simulink model "weight_update"  (R2020a)
settings: Solver=VariableStepAuto  StartTime=0.0  StopTime=6  RelTol=1e-3
libraries: fl_lib x23, ee_lib x10, nesl_utility x7
settings Model: Creator=nick  LastModifiedBy=nick

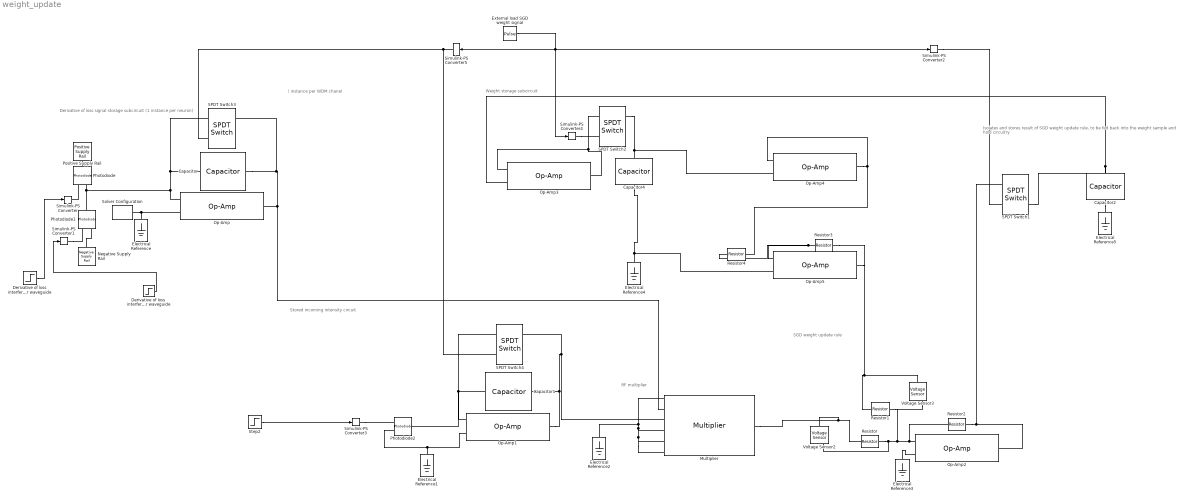
== system weight_update ==
  note: Stored incoming intensity circuit
  note: Derivative of loss signal storage subcircuit
      | (1 instance per neuron)
  note: Weight storage subcircuit
  note: RF multiplier
  note: SGD weight update rule
  note: Isolates and stores result of SGD weight update rule, to be fed back into the weight sample and hold circuitry
  note: ! instance per WDM chanel
  Capacitor : fl_lib/Electrical/Electrical Elements/Capacitor  c=1e-6 F  r=1e-6 Ohm  g=0 1/Ohm  i_specify=off  i_priority=None  i=0 A  i_nominal_specify=off  i_nominal_unit=A  i_nominal_value=1  v_specify=off  v_priority=None  v=0 V  v_nominal_specify=off  v_nominal_unit=V  v_nominal_value=1  vc_specify=off  vc_priority=High  vc=0 V  vc_nominal_specify=off  vc_nominal_unit=V  vc_nominal_value=1
  Capacitor1 : fl_lib/Electrical/Electrical Elements/Capacitor  c=1e-6 F  r=1e-6 Ohm  g=0 1/Ohm  i_specify=off  i_priority=None  i=0 A  i_nominal_specify=off  i_nominal_unit=A  i_nominal_value=1  v_specify=off  v_priority=None  v=0 V  v_nominal_specify=off  v_nominal_unit=V  v_nominal_value=1  vc_specify=off  vc_priority=High  vc=0 V  vc_nominal_specify=off  vc_nominal_unit=V  vc_nominal_value=1
  Capacitor2 : fl_lib/Electrical/Electrical Elements/Capacitor  c=1e-6 F  r=1e-6 Ohm  g=0 1/Ohm  i_specify=off  i_priority=None  i=0 A  i_nominal_specify=off  i_nominal_unit=A  i_nominal_value=1  v_specify=off  v_priority=None  v=0 V  v_nominal_specify=off  v_nominal_unit=V  v_nominal_value=1  vc_specify=on  vc_priority=High  vc=0 V  vc_nominal_specify=off  vc_nominal_unit=V  vc_nominal_value=1
  Capacitor4 : fl_lib/Electrical/Electrical Elements/Capacitor  c=1e-6 F  r=1e-6 Ohm  g=0 1/Ohm  i_specify=off  i_priority=None  i=0 A  i_nominal_specify=off  i_nominal_unit=A  i_nominal_value=1  v_specify=off  v_priority=None  v=0 V  v_nominal_specify=off  v_nominal_unit=V  v_nominal_value=1  vc_specify=on  vc_priority=High  vc=2.5 V  vc_nominal_specify=off  vc_nominal_unit=V  vc_nominal_value=1
  Derivative of loss interfered with 180 degree phase delayed power waveguide : Step  Time=0.5  SampleTime=0.5
  Derivative of loss interfered with power waveguide : Step  Time=0.5  After=2  SampleTime=0.5
  Electrical Reference{,1..5} (6 alike) : fl_lib/Electrical/Electrical Elements/Electrical Reference
  External load SGD weight signal : DiscretePulseGenerator  PulseType=Time based  Period=3  PulseWidth=.5  PhaseDelay=2
  Multiplier : ee_lib/Integrated Circuits/Multiplier  K=10 V  A=3000  Rin=10e6 Ohm  Vdiff=10 V  Rout=0.1 Ohm  Vmin=-11 V  Vmax=11 V  Vdotmax=20 V/us  f=1 MHz  V0=0 V
      settings: SourceProductBaseCode=PS  InternalSimscapePortConfiguration="{\"Bottom\":[],\"Left\":[{\"id\":\"X1\",\"label\":\"X1\",\"type\":\"foundation.electrical.electrical\"},{\"id\":\"X2\",\"label\":\"X2\",\"type\":\"foundation.electrical.electrical\"},{\"id\":\"Y1\",\"label\":\"Y1\",\"type\":\"foundation.electrical.electrical\"},{\"id\":\"Y2\",\"label\":\"Y2\",\"type\":\"foundation.electrical.electrical\"},{\"id\":\"Z1\",\"label\":\"Z1\",\"type\":\"foundation.electrical.electrical\"},{\"id\":\"Z2\",\"label\":\"Z2\",\"type\":\"foundation.electrical.electrical\"}],\"Right\":[{\"id\":\"out\",\"label\":\"\",\"type\":\"foundation.electrical.electrical\"}],\"Top\":[]}"
  Negative Supply Rail : ee_lib/Sources/Negative Supply Rail  v0=-1 V
      settings: SourceProductBaseCode=PS  InternalSimscapePortConfiguration="{\"Bottom\":[],\"Left\":[{\"id\":\"n\",\"label\":\"\",\"type\":\"foundation.electrical.electrical\"}],\"Right\":[],\"Top\":[]}"
  Op-Amp{,1..5} (6 alike) : fl_lib/Electrical/Electrical Elements/Op-Amp  outI_specify=off  outI_priority=None  outI=0 A  outI_nominal_specify=off  outI_nominal_unit=A  outI_nominal_value=1
  Photodiode : ee_lib/Sensors & Transducers/Photodiode  prmFlux=2  Imeas=1 uA  FluxD=5 W/m^2  G=1e-6 m^2*A/W  prmExp=1  I2=0.1 A  V2=1.3 V  IS=5e-9 A  ec=3  RS=0.1 Ohm  Tmeas=25 degC  C_param=1  CJ=60 pF  CJ0=60 pF  VJ=1 V  Mgrad=0.5  Vvec=[.1, 10, 100] V  Cvec=[45, 3, 6] pF  FC=0.5  T_param=1  IS_T2=2.5e-7 A  I1_T2=0.07 A  V1_T2=1.3 V  Tmeas2=125 degC  EG_param=1  EG=1.11 eV  XTI_param=1  XTI=3  Tdevice=25 degC  i_capacitor_specify=off  i_capacitor_priority=High  i_capacitor=0 A  i_capacitor_nominal_specify=off  i_capacitor_nominal_unit=A  i_capacitor_nominal_value=1  v_capacitor_specify=off  v_capacitor_priority=None  v_capacitor=0 V  v_capacitor_nominal_specify=off  v_capacitor_nominal_unit=V  v_capacitor_nominal_value=1  thermal_network_parameterization=ee.enum.thermalNetworkTopology.cauer  Rth=[0, 10] K/W  Rth_Foster=[4, 6] K/W  thermal_mass_parameterization=ee.enum.thermalNetwork.timeconstant  thermal_mass=[0, 1] J/K  thermal_mass_Foster=[1.5, 3] J/K  thermal_time_constant=[0, 10] s  thermal_time_constant_Foster=[6, 18] s  thermal_mass_initial_temperatures=[25, 25] degC
      settings: SourceProductBaseCode=PS  InternalSimscapePortConfiguration="{\"Bottom\":[],\"Left\":[{\"id\":\"W\",\"label\":\"W\",\"type\":\"input\"},{\"id\":\"p\",\"label\":\"\",\"type\":\"foundation.electrical.electrical\"}],\"Right\":[{\"id\":\"n\",\"label\":\"\",\"type\":\"foundation.electrical.electrical\"}],\"Top\":[]}"
  Photodiode1 : ee_lib/Sensors & Transducers/Photodiode  prmFlux=2  Imeas=1 uA  FluxD=5 W/m^2  G=1e-6 m^2*A/W  prmExp=1  I2=0.1 A  V2=1.3 V  IS=5e-9 A  ec=3  RS=0.1 Ohm  Tmeas=25 degC  C_param=1  CJ=60 pF  CJ0=60 pF  VJ=1 V  Mgrad=0.5  Vvec=[.1, 10, 100] V  Cvec=[45, 3, 6] pF  FC=0.5  T_param=1  IS_T2=2.5e-7 A  I1_T2=0.07 A  V1_T2=1.3 V  Tmeas2=125 degC  EG_param=1  EG=1.11 eV  XTI_param=1  XTI=3  Tdevice=25 degC  i_capacitor_specify=off  i_capacitor_priority=High  i_capacitor=0 A  i_capacitor_nominal_specify=off  i_capacitor_nominal_unit=A  i_capacitor_nominal_value=1  v_capacitor_specify=off  v_capacitor_priority=None  v_capacitor=0 V  v_capacitor_nominal_specify=off  v_capacitor_nominal_unit=V  v_capacitor_nominal_value=1  thermal_network_parameterization=ee.enum.thermalNetworkTopology.cauer  Rth=[0, 10] K/W  Rth_Foster=[4, 6] K/W  thermal_mass_parameterization=ee.enum.thermalNetwork.timeconstant  thermal_mass=[0, 1] J/K  thermal_mass_Foster=[1.5, 3] J/K  thermal_time_constant=[0, 10] s  thermal_time_constant_Foster=[6, 18] s  thermal_mass_initial_temperatures=[25, 25] degC
      settings: SourceProductBaseCode=PS  InternalSimscapePortConfiguration="{\"Bottom\":[],\"Left\":[{\"id\":\"W\",\"label\":\"W\",\"type\":\"input\"},{\"id\":\"p\",\"label\":\"\",\"type\":\"foundation.electrical.electrical\"}],\"Right\":[{\"id\":\"n\",\"label\":\"\",\"type\":\"foundation.electrical.electrical\"}],\"Top\":[]}"
  Photodiode2 : ee_lib/Sensors & Transducers/Photodiode  prmFlux=2  Imeas=1 uA  FluxD=5 W/m^2  G=1e-6 m^2*A/W  prmExp=1  I2=0.1 A  V2=1.3 V  IS=5e-9 A  ec=3  RS=0.1 Ohm  Tmeas=25 degC  C_param=1  CJ=60 pF  CJ0=60 pF  VJ=1 V  Mgrad=0.5  Vvec=[.1, 10, 100] V  Cvec=[45, 3, 6] pF  FC=0.5  T_param=1  IS_T2=2.5e-7 A  I1_T2=0.07 A  V1_T2=1.3 V  Tmeas2=125 degC  EG_param=1  EG=1.11 eV  XTI_param=1  XTI=3  Tdevice=25 degC  i_capacitor_specify=off  i_capacitor_priority=High  i_capacitor=0 A  i_capacitor_nominal_specify=off  i_capacitor_nominal_unit=A  i_capacitor_nominal_value=1  v_capacitor_specify=off  v_capacitor_priority=None  v_capacitor=0 V  v_capacitor_nominal_specify=off  v_capacitor_nominal_unit=V  v_capacitor_nominal_value=1  thermal_network_parameterization=ee.enum.thermalNetworkTopology.cauer  Rth=[0, 10] K/W  Rth_Foster=[4, 6] K/W  thermal_mass_parameterization=ee.enum.thermalNetwork.timeconstant  thermal_mass=[0, 1] J/K  thermal_mass_Foster=[1.5, 3] J/K  thermal_time_constant=[0, 10] s  thermal_time_constant_Foster=[6, 18] s  thermal_mass_initial_temperatures=[25, 25] degC
      settings: SourceProductBaseCode=PS  InternalSimscapePortConfiguration="{\"Bottom\":[],\"Left\":[{\"id\":\"W\",\"label\":\"W\",\"type\":\"input\"},{\"id\":\"p\",\"label\":\"\",\"type\":\"foundation.electrical.electrical\"}],\"Right\":[{\"id\":\"n\",\"label\":\"\",\"type\":\"foundation.electrical.electrical\"}],\"Top\":[]}"
  Positive Supply Rail : ee_lib/Sources/Positive Supply Rail  v0=1 V
      settings: SourceProductBaseCode=PS  InternalSimscapePortConfiguration="{\"Bottom\":[],\"Left\":[],\"Right\":[{\"id\":\"p\",\"label\":\"\",\"type\":\"foundation.electrical.electrical\"}],\"Top\":[]}"
  Resistor{,1..4} (5 alike) : fl_lib/Electrical/Electrical Elements/Resistor  R=1 Ohm  i_specify=off  i_priority=None  i=0 A  i_nominal_specify=off  i_nominal_unit=A  i_nominal_value=1  v_specify=off  v_priority=None  v=0 V  v_nominal_specify=off  v_nominal_unit=V  v_nominal_value=1
  SPDT Switch{1..4} (4 alike) : ee_lib/Switches & Breakers/SPDT Switch  R_closed=0.01 Ohm  G_open=1 nS  Threshold=0.5 V  Width=0 V  model_dynamics=0  t_on=1e-3 s  t_off=1e-3 s  initial_vT=0 V
      settings: SourceProductBaseCode=PS
  Simulink-PS Converter{,1..5} (6 alike) : nesl_utility/Simulink-PS Converter  PhysicalDomain=network_engine_domain  SubClassName=ps_input  LeftPortType=input  RightPortType=output  PseudoPeriodic=off  Frequencies=[]  NoiseDistribution=none  NoiseParameters=[]  Unit=1  AffineConversion=off  FilteringAndDerivatives=provide  SimscapeFilterOrder=1  InputFilterTimeConstant=0.001  UdotUserProvided=0
  Solver Configuration : nesl_utility/Solver Configuration  PhysicalDomain=network_engine_domain  SubClassName=solver  LeftPortType=input  RightPortType=generic  Tones=[]  Harmonics=[]  SimulateNoise=off  Profile=off  UseLocalSampling=off  EnableSwitchedLinearOptims=on  FrequencyDomain=off  UseCCode=off  RelTol=0.001  AbsTol=1e-06  MinStep=1e-09  ToWorkspace=off  RevertToSquareIcSolve=off  NumHomotopyIterations=100  PhasorMode=off  PhasorModeNumHarmonics=1  DoDC=off  ResidualTolerance=1e-09  UseLocalSolver=off  LocalSolverChoice=NE_BACKWARD_EULER_ADVANCER  LocalSolverSampleTime=0.001  DoFixedCost=off  MaxNonlinIter=3  MaxModeIter=2  LinearAlgebra=auto  EquationFormulation=NE_TIME_EF  DelaysMemoryBudget=1024  AutomaticFiltering=on  FilteringTimeConstant=0.001  PartitionStorageMethod=AS_NEEDED  PartitionMemoryBudget=1024  PartitionMethod=ROBUST
  Step2 : Step  Time=0.5  After=5  SampleTime=0.5
  Voltage Sensor2 : fl_lib/Electrical/Electrical Sensors/Voltage Sensor
  Voltage Sensor3 : fl_lib/Electrical/Electrical Sensors/Voltage Sensor
  wires:
  Derivative of loss interfered with power waveguide/1 -> Simulink-PS Converter/1
  Derivative of loss interfered with 180 degree phase delayed power waveguide/1 -> Simulink-PS Converter1/1
  Step2/1 -> Simulink-PS Converter3/1
  External load SGD weight signal/1 -> Simulink-PS Converter4/1, Simulink-PS Converter2/1, Simulink-PS Converter5/1
  connections:
  Capacitor/RConn1 -- SPDT Switch3/RConn2 -- Multiplier/LConn2 -- Op-Amp/RConn1
  Electrical Reference/LConn1 -- Solver Configuration/RConn1 -- Op-Amp/LConn1
  Photodiode/LConn2 -- Op-Amp/LConn2 -- SPDT Switch3/LConn2 -- Capacitor/LConn1 -- Photodiode1/RConn1
  Positive Supply Rail/RConn1 -- Photodiode/RConn1
  Negative Supply Rail/LConn1 -- Photodiode1/LConn2
  Simulink-PS Converter1/RConn1 -- Photodiode1/LConn1
  Simulink-PS Converter/RConn1 -- Photodiode/LConn1
  Photodiode2/LConn2 -- Electrical Reference1/LConn1 -- Op-Amp1/LConn1
  Op-Amp1/RConn1 -- SPDT Switch4/RConn2 -- Multiplier/LConn3 -- Capacitor1/RConn1
  Simulink-PS Converter3/RConn1 -- Photodiode2/LConn1
  Photodiode2/RConn1 -- Op-Amp1/LConn2 -- SPDT Switch4/LConn2 -- Capacitor1/LConn1
  Electrical Reference2/LConn1 -- Multiplier/LConn1 -- Multiplier/LConn6 -- Multiplier/LConn5 -- Multiplier/LConn4
  Multiplier/RConn1 -- Resistor/LConn1 -- Voltage Sensor2/LConn1
  Resistor/RConn1 -- Voltage Sensor2/RConn2 -- Voltage Sensor3/RConn2 -- Resistor1/RConn1 -- Resistor2/LConn1 -- Op-Amp2/LConn2
  Electrical Reference3/LConn1 -- Op-Amp2/LConn1
  Resistor3/RConn1 -- Op-Amp5/RConn1 -- Resistor1/LConn1 -- Voltage Sensor3/LConn1
  Resistor2/RConn1 -- Op-Amp2/RConn1 -- SPDT Switch1/LConn2
  Capacitor2/RConn1 -- Electrical Reference5/LConn1
  SPDT Switch1/RConn1 -- Op-Amp3/LConn1 -- Capacitor2/LConn1
  Simulink-PS Converter2/RConn1 -- SPDT Switch1/LConn1
  Op-Amp3/LConn2 -- Op-Amp3/RConn1 -- SPDT Switch2/LConn2
  SPDT Switch2/RConn2 -- Capacitor4/LConn1 -- Op-Amp4/LConn1
  Electrical Reference4/LConn1 -- Capacitor4/RConn1 -- Op-Amp5/LConn1
  Simulink-PS Converter4/RConn1 -- SPDT Switch2/LConn1
  Resistor3/LConn1 -- Resistor4/LConn1 -- Op-Amp5/LConn2
  Op-Amp4/RConn1 -- Resistor4/RConn1 -- Op-Amp4/LConn2
  Simulink-PS Converter5/RConn1 -- SPDT Switch4/LConn1 -- SPDT Switch3/LConn1
